simulink model "model3part2"  (R2018b)
settings: Solver=ode4  StartTime=0.0  StopTime=10.0  FixedStep=0.01  RelTol=1e-3
values from neighbouring files (symbols this model uses):
  gd1 = g21    [script3.m]
  gd2 = g22    [script3.m]
settings Model: Creator=Joanna  LastModifiedBy=Joanna

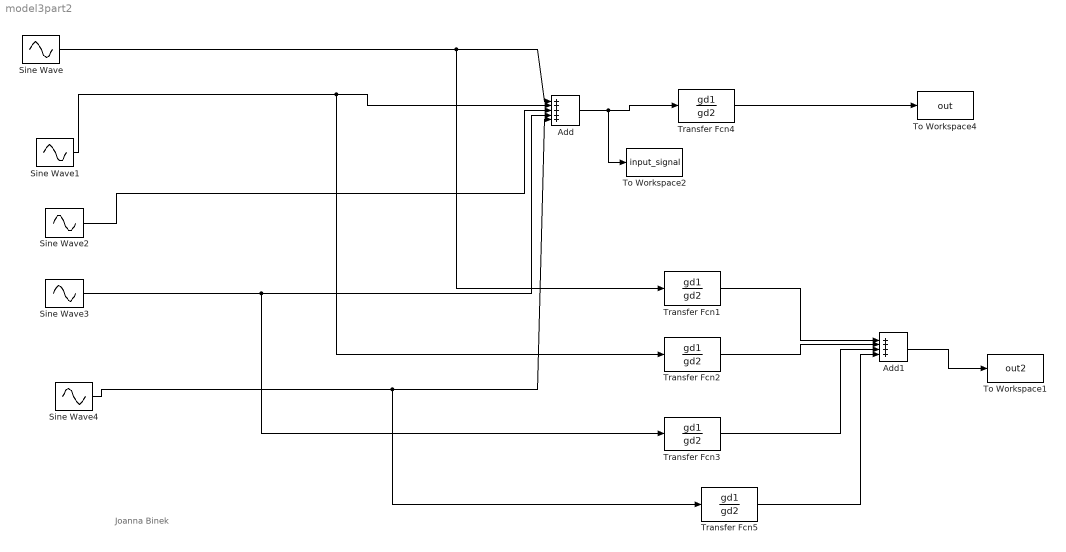
== system model3part2 ==
  note: Joanna Binek
  Add : Sum  Inputs=+++++
  Add1 : Sum  Inputs=++++
  Sine Wave : Sin  Amplitude=2  Frequency=0.001  Phase=1  SampleTime=0
  Sine Wave1 : Sin  Amplitude=3  Phase=5  SampleTime=0
  Sine Wave2 : Sin  Frequency=30  Phase=2  SampleTime=0
  Sine Wave3 : Sin  Amplitude=2  Frequency=0.01  Phase=1  SampleTime=0
  Sine Wave4 : Sin  Amplitude=4  Frequency=5  SampleTime=0
  To Workspace1 : ToWorkspace  VariableName=out2  SampleTime=-1
  To Workspace2 : ToWorkspace  VariableName=input_signal  SampleTime=-1
  To Workspace4 : ToWorkspace  VariableName=out  SampleTime=-1
  Transfer Fcn{1..5} (5 alike) : TransferFcn  Numerator=gd1  Denominator=gd2
  wires:
  Add/1 -> To Workspace2/1, Transfer Fcn4/1
  Sine Wave/1 -> Transfer Fcn1/1, Add/1
  Sine Wave3/1 -> Transfer Fcn3/1, Add/4
  Sine Wave2/1 -> Add/3
  Sine Wave4/1 -> Transfer Fcn5/1, Add/5
  Transfer Fcn4/1 -> To Workspace4/1
  Sine Wave1/1 -> Transfer Fcn2/1, Add/2
  Transfer Fcn1/1 -> Add1/1
  Transfer Fcn2/1 -> Add1/2
  Transfer Fcn3/1 -> Add1/3
  Transfer Fcn5/1 -> Add1/4
  Add1/1 -> To Workspace1/1
